simulink model "sixth_10_03_25class_partB"  (R2024a)
settings: Solver=VariableStepAuto  StartTime=0.0  StopTime=inf  MaxStep=1e-6  RelTol=1e-3
undefined symbols (not defined in the file): fsw, l, r
libraries: simulink x3
settings Model: Creator=claudio.rossi  LastModifiedBy=s0001205361
settings OptimizationCC: ReuseModelBlockBuffer=off
settings RTWCC: GPUComputeCapability=3.5

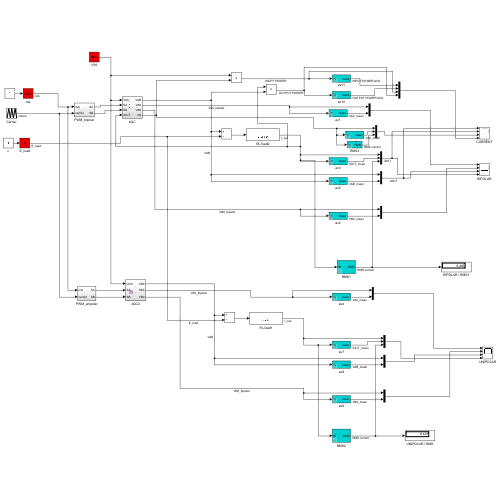
[thumbnail: Simulink's stored preview of the top-level diagram]
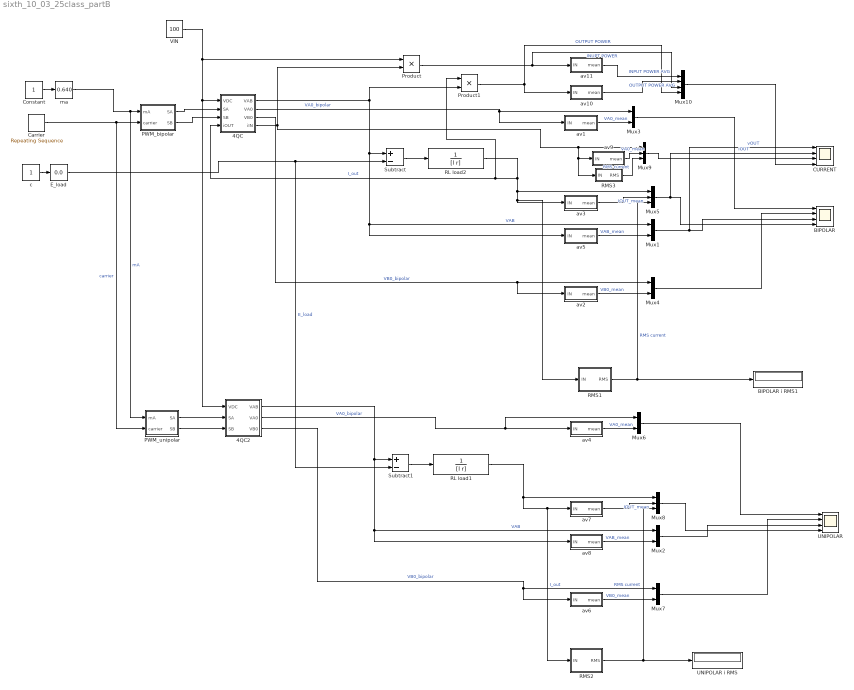
== system sixth_10_03_25class_partB ==
  4QC : Subsystem
  4QC2 : Subsystem
  BIPOLAR : Scope  NumInputPorts=4
  BIPOLAR i RMS1 : Display
  CURRENT : Scope  NumInputPorts=4
  "Carrier " : simulink/Sources/Repeating Sequence  rep_seq_t=[0 0.5/fsw 1/fsw]  rep_seq_y=[-1 1 -1 ]
  Constant : Constant
  E_load : simulink/Math Operations/Slider Gain  gain=0.0  low=0  high=200
  Mux{1..4,6..7} (6 alike) : Mux  Inputs=2
  Mux10 : Mux
  Mux5 : Mux  Inputs=3
  Mux8 : Mux  Inputs=3
  Mux9 : Mux  Inputs=3
  PWM_bipolar : Subsystem
  PWM_unipolar : Subsystem
  Product : Product
  Product1 : Product
  RL load1 : TransferFcn  Denominator=[l r]
  RL load2 : TransferFcn  Denominator=[l r]
  RMS1 : Subsystem  mask{period=20e-3}
      mask prompts: period "period [s]"
      mask DialogControl DescTextVar Prompt: calculates the RMS of a periodic function with period specified here
  RMS2 : Subsystem  mask{period=20e-3}
      mask prompts: period "period [s]"
      mask DialogControl DescTextVar Prompt: calculates the RMS of a periodic function with period specified here
  RMS3 : Subsystem  mask{period=20e-3}
      mask prompts: period "period [s]"
      mask DialogControl DescTextVar Prompt: calculates the RMS of a periodic function with period specified here
  Subtract : Sum  Inputs=+-
  Subtract1 : Sum  Inputs=+-
  UNIPOLAR : Scope  NumInputPorts=4
  UNIPOLAR i RMS : Display
  VIN : Constant  Value=100
  av1 : Subsystem  mask{period=1/fsw}
      mask prompts: period "period [s]"
      mask DialogControl DescTextVar Prompt: calculate the averge over period
      mask DialogControl text Prompt: test
  av10 : Subsystem  mask{period=1/fsw}
      mask prompts: period "period [s]"
      mask DialogControl DescTextVar Prompt: calculate the averge over period
      mask DialogControl text Prompt: test
  av11 : Subsystem  mask{period=1/fsw}
      mask prompts: period "period [s]"
      mask DialogControl DescTextVar Prompt: calculate the averge over period
      mask DialogControl text Prompt: test
  av2 : Subsystem  mask{period=1/fsw}
      mask prompts: period "period [s]"
      mask DialogControl DescTextVar Prompt: calculate the averge over period
      mask DialogControl text Prompt: test
  av3 : Subsystem  mask{period=1/fsw}
      mask prompts: period "period [s]"
      mask DialogControl DescTextVar Prompt: calculate the averge over period
      mask DialogControl text Prompt: test
  av4 : Subsystem  mask{period=1/fsw}
      mask prompts: period "period [s]"
      mask DialogControl DescTextVar Prompt: calculate the averge over period
      mask DialogControl text Prompt: test
  av5 : Subsystem  mask{period=1/fsw}
      mask prompts: period "period [s]"
      mask DialogControl DescTextVar Prompt: calculate the averge over period
      mask DialogControl text Prompt: test
  av6 : Subsystem  mask{period=1/fsw}
      mask prompts: period "period [s]"
      mask DialogControl DescTextVar Prompt: calculate the averge over period
      mask DialogControl text Prompt: test
  av7 : Subsystem  mask{period=1/fsw}
      mask prompts: period "period [s]"
      mask DialogControl DescTextVar Prompt: calculate the averge over period
      mask DialogControl text Prompt: test
  av8 : Subsystem  mask{period=1/fsw}
      mask prompts: period "period [s]"
      mask DialogControl DescTextVar Prompt: calculate the averge over period
      mask DialogControl text Prompt: test
  av9 : Subsystem  mask{period=1/fsw}
      mask prompts: period "period [s]"
      mask DialogControl DescTextVar Prompt: calculate the averge over period
      mask DialogControl text Prompt: test
  c : Constant
  ma : simulink/Math Operations/Slider Gain  gain=0.640  low=-1  high=1
  wires:
  ma/1 -> PWM_unipolar/1(mA), PWM_bipolar/1(mA)  "mA"
  Constant/1 -> ma/1
  4QC/1(VAB) -> av5/1(IN), Mux1/1, Subtract/1, Product1/2  "VAB"
  c/1 -> E_load/1
  Subtract/1 -> RL load2/1
  av5/1(mean) -> Mux1/2  "VAB_mean"
  Mux1/1 -> CURRENT/1, BIPOLAR/3  "vOUT"
  Mux3/1 -> BIPOLAR/1
  av1/1(mean) -> Mux3/2  "VA0_mean"
  av2/1(mean) -> Mux4/2  "VB0_mean"
  Mux4/1 -> BIPOLAR/2
  Mux5/1 -> CURRENT/2, BIPOLAR/4  "iOUT"
  av3/1(mean) -> Mux5/2  "IOUT_mean"
  RL load2/1 -> Product1/1, 4QC/4(iOUT), Mux5/1, RMS1/1(IN), av3/1(IN)  "I_out"
  PWM_bipolar/1(SA) -> 4QC/2(SA)
  PWM_bipolar/2(SB) -> 4QC/3(SB)
  "Carrier "/1 -> PWM_unipolar/2(carrier), PWM_bipolar/2(carrier)  "carrier"
  VIN/1 -> 4QC2/1(VDC), 4QC/1(VDC), Product/1
  4QC/2(VA0) -> av1/1(IN), Mux3/1  "VA0_bipolar"
  PWM_unipolar/1(SA) -> 4QC2/2(SA)
  PWM_unipolar/2(SB) -> 4QC2/3(SB)
  4QC/3(VB0) -> av2/1(IN), Mux4/1  "VB0_bipolar"
  4QC2/3(VB0) -> Mux7/1, av6/1(IN)  "VB0_bipolar"
  4QC2/2(VA0) -> av4/1(IN), Mux6/1  "VA0_bipolar"
  RL load1/1 -> RMS2/1(IN), av7/1(IN), Mux8/1  "I_out"
  av7/1(mean) -> Mux8/2  "IOUT_mean"
  Mux8/1 -> UNIPOLAR/4
  Mux7/1 -> UNIPOLAR/2
  av6/1(mean) -> Mux7/2  "VB0_mean"
  av4/1(mean) -> Mux6/2  "VA0_mean"
  Mux6/1 -> UNIPOLAR/1
  Mux2/1 -> UNIPOLAR/3
  av8/1(mean) -> Mux2/2  "VAB_mean"
  Subtract1/1 -> RL load1/1
  E_load/1 -> Subtract1/2, Subtract/2  "E_load"
  4QC2/1(VAB) -> Subtract1/1, Mux2/1, av8/1(IN)  "VAB"
  RMS2/1(RMS) -> Mux8/3, UNIPOLAR i RMS/1  "RMS current"
  RMS1/1(RMS) -> Mux5/3, BIPOLAR i RMS1/1  "RMS current"
  4QC/4(iIN) -> Product/2, Mux9/1, RMS3/1(IN), av9/1(IN)
  av9/1(mean) -> Mux9/2  "VA0_mean"
  Mux9/1 -> CURRENT/3
  RMS3/1(RMS) -> Mux9/3  "RMS current"
  Product1/1 -> Mux10/4, av10/1(IN)  "OUTPUT POWER"
  Product/1 -> Mux10/3, av11/1(IN)  "INUPT POWER"
  av11/1(mean) -> Mux10/1  "INPUT POWER AVG"
  av10/1(mean) -> Mux10/2  "OUTPUT POWER AVG"
  Mux10/1 -> CURRENT/4

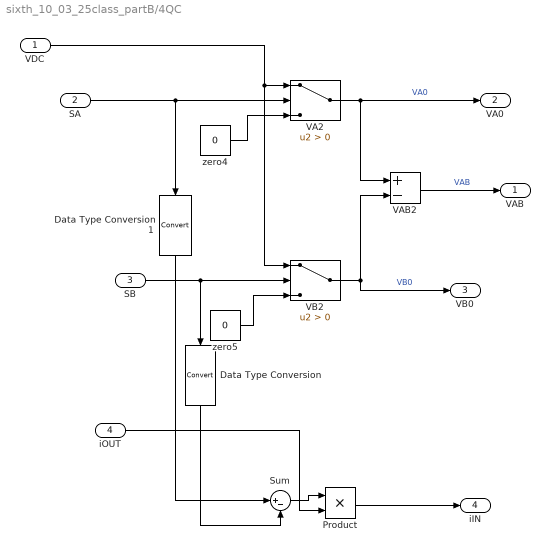
== system sixth_10_03_25class_partB/4QC ==
  VDC : Inport
  SA : Inport  Port=2
  SB : Inport  Port=3
  iOUT : Inport  Port=4
  Data Type Conversion : DataTypeConversion  SaturateOnIntegerOverflow=off  RndMeth=Floor
  Data Type Conversion1 : DataTypeConversion  SaturateOnIntegerOverflow=off  RndMeth=Floor
  Product : Product
  Sum : Sum  Inputs=|+-
  VA2 : Switch  Criteria=u2 > Threshold  SaturateOnIntegerOverflow=off  InputSameDT=off
  VAB2 : Sum  Inputs=+-
  VB2 : Switch  Criteria=u2 > Threshold  SaturateOnIntegerOverflow=off  InputSameDT=off
  zero4 : Constant  Value=0
  zero5 : Constant  Value=0
  VAB : Outport
  VA0 : Outport  Port=2
  VB0 : Outport  Port=3
  iIN : Outport  Port=4
  wires:
  zero5/1 -> VB2/3
  SB/1 -> Data Type Conversion/1, VB2/2
  zero4/1 -> VA2/3
  VDC/1 -> VA2/1, VB2/1
  SA/1 -> VA2/2, Data Type Conversion1/1
  VA2/1 -> VA0/1, VAB2/1  "VA0"
  VAB2/1 -> VAB/1  "VAB"
  VB2/1 -> VAB2/2, VB0/1  "VB0"
  Sum/1 -> Product/1
  Product/1 -> iIN/1
  iOUT/1 -> Product/2
  Data Type Conversion1/1 -> Sum/1
  Data Type Conversion/1 -> Sum/2

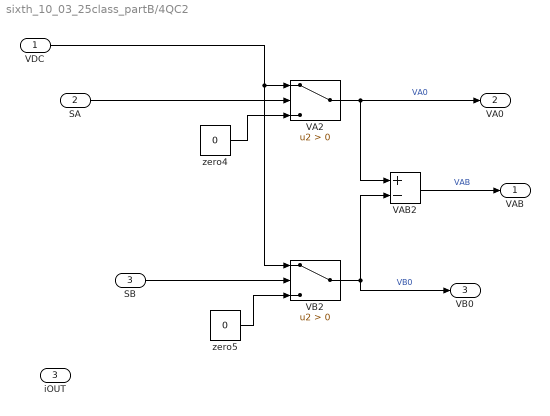
== system sixth_10_03_25class_partB/4QC2 ==
  VDC : Inport
  SA : Inport  Port=2
  SB : Inport  Port=3
  VA2 : Switch  Criteria=u2 > Threshold  SaturateOnIntegerOverflow=off  InputSameDT=off
  VAB2 : Sum  Inputs=+-
  VB2 : Switch  Criteria=u2 > Threshold  SaturateOnIntegerOverflow=off  InputSameDT=off
  iOUT : InportShadow  Port=3
  zero4 : Constant  Value=0
  zero5 : Constant  Value=0
  VAB : Outport
  VA0 : Outport  Port=2
  VB0 : Outport  Port=3
  wires:
  VB2/1 -> VB0/1, VAB2/2  "VB0"
  VAB2/1 -> VAB/1  "VAB"
  VA2/1 -> VAB2/1, VA0/1  "VA0"
  SA/1 -> VA2/2
  VDC/1 -> VB2/1, VA2/1
  zero4/1 -> VA2/3
  SB/1 -> VB2/2
  zero5/1 -> VB2/3

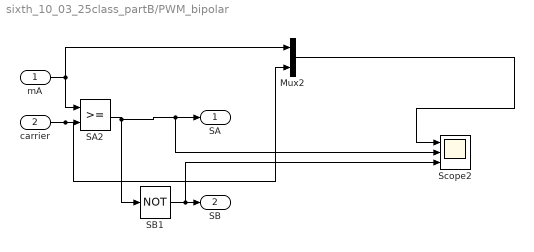
== system sixth_10_03_25class_partB/PWM_bipolar ==
  mA : Inport
  carrier : Inport  Port=2
  Mux2 : Mux  Inputs=2
  SA2 : RelationalOperator  OutDataTypeStr=boolean  RndMeth=Simplest  InputSameDT=off
  SB1 : Logic  Operator=NOT  AllPortsSameDT=off  OutDataTypeStr=boolean
  Scope2 : Scope  NumInputPorts=3
  SA : Outport
  SB : Outport  Port=2
  wires:
  SB1/1 -> SB/1, Scope2/3
  Mux2/1 -> Scope2/1
  SA2/1 -> SB1/1, SA/1, Scope2/2
  carrier/1 -> SA2/2, Mux2/2
  mA/1 -> Mux2/1, SA2/1

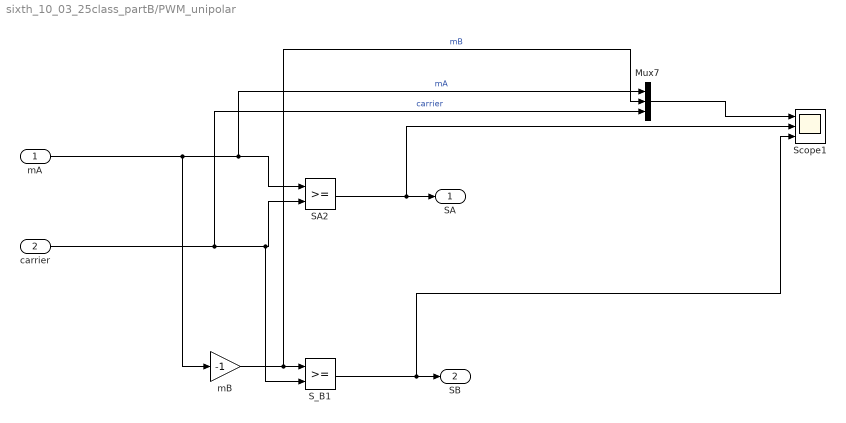
== system sixth_10_03_25class_partB/PWM_unipolar ==
  mA : Inport
  carrier : Inport  Port=2
  Mux7 : Mux  Inputs=3
  SA2 : RelationalOperator  OutDataTypeStr=boolean  RndMeth=Simplest  InputSameDT=off
  S_B1 : RelationalOperator  OutDataTypeStr=boolean  RndMeth=Simplest  InputSameDT=off
  Scope1 : Scope  NumInputPorts=3
  mB : Gain  Gain=-1
  SA : Outport
  SB : Outport  Port=2
  wires:
  mA/1 -> SA2/1, Mux7/1, mB/1  "mA"
  Mux7/1 -> Scope1/1
  SA2/1 -> SA/1, Scope1/2
  S_B1/1 -> SB/1, Scope1/3
  carrier/1 -> SA2/2, S_B1/2, Mux7/3  "carrier"
  mB/1 -> S_B1/1, Mux7/2  "mB"

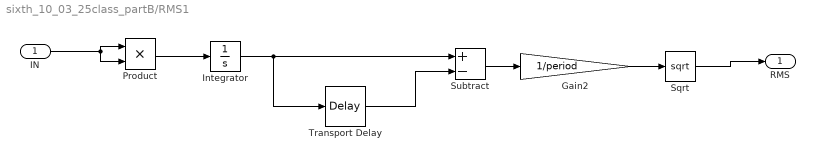
== system sixth_10_03_25class_partB/RMS1 ==
  IN : Inport
  Gain2 : Gain  Gain=1/period
  Integrator : Integrator
  Product : Product
  Sqrt : Sqrt
  Subtract : Sum  Inputs=+-
  Transport Delay : TransportDelay  DelayTime=period
  RMS : Outport
  wires:
  Sqrt/1 -> RMS/1
  Gain2/1 -> Sqrt/1
  Product/1 -> Integrator/1
  IN/1 -> Product/2, Product/1
  Integrator/1 -> Transport Delay/1, Subtract/1
  Subtract/1 -> Gain2/1
  Transport Delay/1 -> Subtract/2

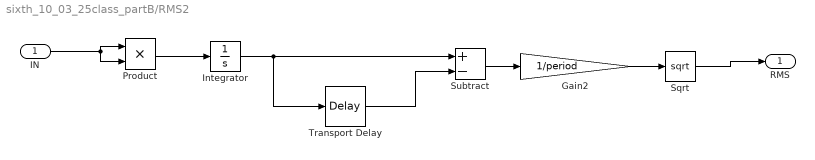
== system sixth_10_03_25class_partB/RMS2 ==
  IN : Inport
  Gain2 : Gain  Gain=1/period
  Integrator : Integrator
  Product : Product
  Sqrt : Sqrt
  Subtract : Sum  Inputs=+-
  Transport Delay : TransportDelay  DelayTime=period
  RMS : Outport
  wires:
  Transport Delay/1 -> Subtract/2
  Subtract/1 -> Gain2/1
  Integrator/1 -> Subtract/1, Transport Delay/1
  IN/1 -> Product/1, Product/2
  Product/1 -> Integrator/1
  Gain2/1 -> Sqrt/1
  Sqrt/1 -> RMS/1

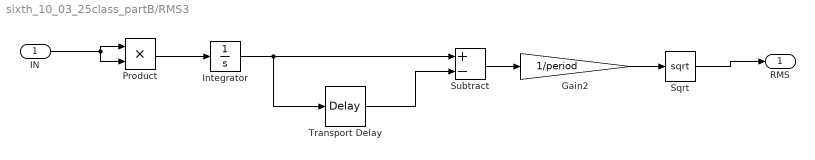
== system sixth_10_03_25class_partB/RMS3 ==
  IN : Inport
  Gain2 : Gain  Gain=1/period
  Integrator : Integrator
  Product : Product
  Sqrt : Sqrt
  Subtract : Sum  Inputs=+-
  Transport Delay : TransportDelay  DelayTime=period
  RMS : Outport
  wires:
  Transport Delay/1 -> Subtract/2
  Subtract/1 -> Gain2/1
  Integrator/1 -> Subtract/1, Transport Delay/1
  IN/1 -> Product/1, Product/2
  Product/1 -> Integrator/1
  Gain2/1 -> Sqrt/1
  Sqrt/1 -> RMS/1

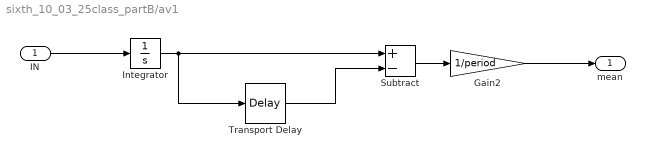
== system sixth_10_03_25class_partB/av1 ==
  IN : Inport
  Gain2 : Gain  Gain=1/period
  Integrator : Integrator
  Subtract : Sum  Inputs=+-
  Transport Delay : TransportDelay  DelayTime=period
  mean : Outport
  wires:
  Integrator/1 -> Transport Delay/1, Subtract/1
  Gain2/1 -> mean/1
  Subtract/1 -> Gain2/1
  Transport Delay/1 -> Subtract/2
  IN/1 -> Integrator/1

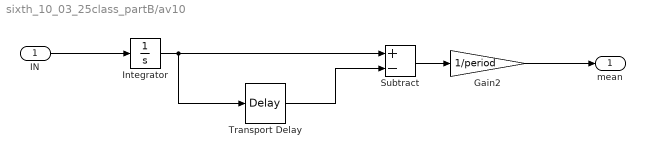
== system sixth_10_03_25class_partB/av10 ==
  IN : Inport
  Gain2 : Gain  Gain=1/period
  Integrator : Integrator
  Subtract : Sum  Inputs=+-
  Transport Delay : TransportDelay  DelayTime=period
  mean : Outport
  wires:
  Integrator/1 -> Transport Delay/1, Subtract/1
  Gain2/1 -> mean/1
  Subtract/1 -> Gain2/1
  Transport Delay/1 -> Subtract/2
  IN/1 -> Integrator/1

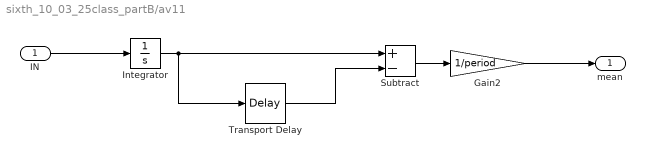
== system sixth_10_03_25class_partB/av11 ==
  IN : Inport
  Gain2 : Gain  Gain=1/period
  Integrator : Integrator
  Subtract : Sum  Inputs=+-
  Transport Delay : TransportDelay  DelayTime=period
  mean : Outport
  wires:
  IN/1 -> Integrator/1
  Transport Delay/1 -> Subtract/2
  Subtract/1 -> Gain2/1
  Gain2/1 -> mean/1
  Integrator/1 -> Subtract/1, Transport Delay/1

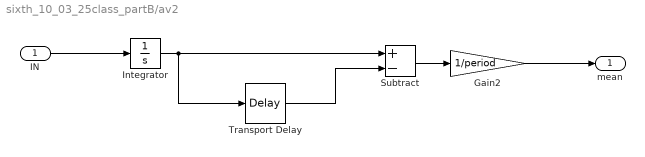
== system sixth_10_03_25class_partB/av2 ==
  IN : Inport
  Gain2 : Gain  Gain=1/period
  Integrator : Integrator
  Subtract : Sum  Inputs=+-
  Transport Delay : TransportDelay  DelayTime=period
  mean : Outport
  wires:
  IN/1 -> Integrator/1
  Transport Delay/1 -> Subtract/2
  Subtract/1 -> Gain2/1
  Gain2/1 -> mean/1
  Integrator/1 -> Subtract/1, Transport Delay/1

== system sixth_10_03_25class_partB/av3 ==
  IN : Inport
  Gain2 : Gain  Gain=1/period
  Integrator : Integrator
  Subtract : Sum  Inputs=+-
  Transport Delay : TransportDelay  DelayTime=period
  mean : Outport
  wires:
  Integrator/1 -> Transport Delay/1, Subtract/1
  Gain2/1 -> mean/1
  Subtract/1 -> Gain2/1
  Transport Delay/1 -> Subtract/2
  IN/1 -> Integrator/1

== system sixth_10_03_25class_partB/av4 ==
  IN : Inport
  Gain2 : Gain  Gain=1/period
  Integrator : Integrator
  Subtract : Sum  Inputs=+-
  Transport Delay : TransportDelay  DelayTime=period
  mean : Outport
  wires:
  IN/1 -> Integrator/1
  Transport Delay/1 -> Subtract/2
  Subtract/1 -> Gain2/1
  Gain2/1 -> mean/1
  Integrator/1 -> Subtract/1, Transport Delay/1

== system sixth_10_03_25class_partB/av5 ==
  IN : Inport
  Gain2 : Gain  Gain=1/period
  Integrator : Integrator
  Subtract : Sum  Inputs=+-
  Transport Delay : TransportDelay  DelayTime=period
  mean : Outport
  wires:
  IN/1 -> Integrator/1
  Transport Delay/1 -> Subtract/2
  Subtract/1 -> Gain2/1
  Gain2/1 -> mean/1
  Integrator/1 -> Subtract/1, Transport Delay/1

== system sixth_10_03_25class_partB/av6 ==
  IN : Inport
  Gain2 : Gain  Gain=1/period
  Integrator : Integrator
  Subtract : Sum  Inputs=+-
  Transport Delay : TransportDelay  DelayTime=period
  mean : Outport
  wires:
  Integrator/1 -> Transport Delay/1, Subtract/1
  Gain2/1 -> mean/1
  Subtract/1 -> Gain2/1
  Transport Delay/1 -> Subtract/2
  IN/1 -> Integrator/1

== system sixth_10_03_25class_partB/av7 ==
  IN : Inport
  Gain2 : Gain  Gain=1/period
  Integrator : Integrator
  Subtract : Sum  Inputs=+-
  Transport Delay : TransportDelay  DelayTime=period
  mean : Outport
  wires:
  IN/1 -> Integrator/1
  Transport Delay/1 -> Subtract/2
  Subtract/1 -> Gain2/1
  Gain2/1 -> mean/1
  Integrator/1 -> Subtract/1, Transport Delay/1

== system sixth_10_03_25class_partB/av8 ==
  IN : Inport
  Gain2 : Gain  Gain=1/period
  Integrator : Integrator
  Subtract : Sum  Inputs=+-
  Transport Delay : TransportDelay  DelayTime=period
  mean : Outport
  wires:
  Integrator/1 -> Transport Delay/1, Subtract/1
  Gain2/1 -> mean/1
  Subtract/1 -> Gain2/1
  Transport Delay/1 -> Subtract/2
  IN/1 -> Integrator/1

== system sixth_10_03_25class_partB/av9 ==
  IN : Inport
  Gain2 : Gain  Gain=1/period
  Integrator : Integrator
  Subtract : Sum  Inputs=+-
  Transport Delay : TransportDelay  DelayTime=period
  mean : Outport
  wires:
  IN/1 -> Integrator/1
  Transport Delay/1 -> Subtract/2
  Subtract/1 -> Gain2/1
  Gain2/1 -> mean/1
  Integrator/1 -> Subtract/1, Transport Delay/1
